simulink model "BaseEngineController_LS"  (Simulink 7.7)
settings: Solver=FixedStepDiscrete  StartTime=0.0  StopTime=10.0  RelTol=1e-3
PreLoadFcn:
  | try, eval([bdroot '_setup']); catch, eval('model_setup', ''); end
InitFcn:
  | try, eval([bdroot '_setup']); catch, eval('model_setup', ''); end
undefined symbols (not defined in the file): ECU555, High, motohawk_build_version, motohawk_trunc_name, motohawk_vardec_config_group, motohawk_vardec_path, True
libraries: MotoHawk_lib x1418, motohawk_control_primitives_lib x183, motohawk_engine_lib x32, simulink x21, motohawk_annotations_lib x9, AutoDoc_lib x8, simulink_extras x4, motohawk_ccp_examples_lib x1, motohawk_control_primitives_motoshare_lib x1
(part 7 of 27)

== system BaseEngineController_LS/Foreground/Control/VirtualSensors/FuelLevel ==
  note: Fuel Level Processed
      | - Detect Refuel Event and immediatly go to new refuled value
      | - If not a refuel event, then filter fuel level at high filter time constant (maybe lower the filter value when vehicle speed is higher), this captures parked on driveway scenario
  Sensors : Inport
  Raw Processed : Inport  Port=2
  Bus Selector : BusSelector  OutputSignals=NonLinearSensors.Fuel_Lvl_Raw
  Bus Selector1 : BusSelector  OutputSignals=TimeSinceKeyOn,VSPD_Final
  First Order Low Pass : motohawk_control_primitives_lib/First Order Low Pass  SystemSampleTime=-1
  FuelLevelWrite : Subsystem  TreatAsAtomicUnit=on
  Logical Operator : Logic  Operator=NOT  AllPortsSameDT=off  OutDataTypeStr=boolean
  Logical Operator1 : Logic  Operator=OR  AllPortsSameDT=off  OutDataTypeStr=boolean
  MinMax : MinMax  Function=max  Inputs=2  SaturateOnIntegerOverflow=on  InputSameDT=on
  Product : Product  Inputs=*/  SaturateOnIntegerOverflow=on  InputSameDT=on  OutDataTypeStr=Inherit: Same as first input
  RefuelEvent : Subsystem
  Switch2 : Switch  Criteria=u2 ~= 0
  Switch3 : Switch  Criteria=u2 ~= 0
  motohawk_calibration2 : MotoHawk_lib/Calibration & Probing Blocks/motohawk_calibration  nam='FuelLevel_FuelEevntAlpha'  val=1  storage=Calibration  show_more=on  name_source=Use Parameter  data_type=Inherit from 'Default Value'  read_level=1  write_level=1  ovr_cals=on  view_as=Number  enum_struct={'Disabled', 'Enabled'}  vector_style=Wide Row  use_help_units=on  help='Fuel event alpha'  units='alpha'  use_header_enum=off  row_header_enum={}  col_header_enum={}  use_min_max=on  min_val=0  max_val=inf  use_precision=off  precision=''  gain=1  offset=0  exp=1  use_mototune_group=off  mototune_group=motohawk_vardec_path(gcb)
  motohawk_data_def : MotoHawk_lib/Data Storage Blocks/motohawk_data_def  nam='FuelLvl_NVM'  container_nam=''  data=0  typ=double  struct_nam='MyStruct'  storage=NonVolatile  outputRef=off  use_vardec=off  window=Calibration  read_level=1  write_level=1  ovr_cals=on  view_as=Number  enum_struct={'Disabled', 'Enabled'}  vector_style=Wide Row  use_help_units=off  help=''  units=''  use_header_enum=off  row_header_enum=''  col_header_enum=''  use_min_max=on  min_val=-inf  max_val=inf  use_precision=off  precision=''  gain=1  offset=0  exp=1  use_mototune_group=off  mototune_group=motohawk_vardec_path(gcb)  eval_name=MyData  data_stores=motohawk_sfun_data_def_data_stores  struct_instances=motohawk_sfun_data_def_struct_instances  vardecs=motohawk_sfun_data_def_vardecs
  motohawk_data_read : MotoHawk_lib/Data Storage Blocks/motohawk_data_read  source=Lookup By Name  structure=Scalar  operation=Read scalar from location by index  sz_vec=4  sz_row=2  sz_col=3  typ=double  nam='FuelLvl_NVM'  checkNull=on  struct_inst_name='MyData'  struct_nam='MyStruct'
  motohawk_delta_time : MotoHawk_lib/Extra Development Blocks/motohawk_delta_time  samp_time=-1  init_val=0  mode=Seconds (double)
  motohawk_probe : MotoHawk_lib/Calibration & Probing Blocks/motohawk_probe  nam='FuelLvl_NVM_Prb'  show_more=off  name_source=Use Parameter  read_level=1  view_as=Number  enum_struct={'Disabled', 'Enabled'}  vector_style=Wide Row  use_help_units=off  help=''  units=''  use_header_enum=off  row_header_enum={}  col_header_enum={}  use_precision=off  precision=''  gain=1  offset=0  exp=1  use_mototune_group=off  mototune_group=motohawk_vardec_path(gcb)
  motohawk_probe1 : MotoHawk_lib/Calibration & Probing Blocks/motohawk_probe  nam='FuelLvl_Fin'  show_more=off  name_source=Use Parameter  read_level=1  view_as=Number  enum_struct={'Disabled', 'Enabled'}  vector_style=Wide Row  use_help_units=off  help=''  units=''  use_header_enum=off  row_header_enum={}  col_header_enum={}  use_precision=off  precision=''  gain=1  offset=0  exp=1  use_mototune_group=off  mototune_group=motohawk_vardec_path(gcb)
  motohawk_table_2d : MotoHawk_lib/Lookup Tables/motohawk_table_2d  SystemSampleTime=-1  nam='FuelLevel_FiltConst'  row_nam=''  col_nam=''  row_breakpoint_data=ones(1,7)  col_breakpoint_data=ones(1,7)  table_data=ones(7)  show_more=on  row_bp_data_type=Inherit from 'Row Breakpoint Data'  col_bp_data_type=Inherit from 'Column Breakpoint Data'  bp_storage=Constant  table_data_type=Inherit from 'Table Data'  storage=NonAdaptive  read_level=1  write_level=1  ovr_cals=on  use_help=on  help='FuelLevel_FiltConst'  row_bp_units='sec'  col_bp_units='mph'  table_units='sec'  use_min_max=on  row_bp_min_val=0  row_bp_max_val=inf  col_bp_min_val=0  col_bp_max_val=inf  min_val=0  max_val=inf  use_precision=off  use_row_breakpoint=off  rb_precision=''  rb_gain=1  rb_offset=0  rb_exp=1  use_col_breakpoint=off  cb_precision=''  cb_gain=1  cb_offset=0  cb_exp=1  use_table=off  t_precision=''  t_gain=1  t_offset=0  t_exp=1  use_links=off  row_input_name=''  col_input_name=''  output_name=''  use_mototune_group=off  mototune_group=motohawk_vardec_path(gcb)
  Fuel Lvl Final : Outport
  wires:
  Sensors/1 -> Bus Selector/1
  Raw Processed/1 -> Bus Selector1/1
  First Order Low Pass/1 -> Fuel Lvl Final/1, motohawk_probe1/1, FuelLevelWrite/1(FuelLevelFilt)
  motohawk_delta_time/1 -> Product/1, MinMax/1
  MinMax/1 -> Product/2
  motohawk_table_2d/1 -> MinMax/2
  Bus Selector1/2 -> motohawk_table_2d/2  "<VSPD_Final>"
  Bus Selector/1 -> RefuelEvent/1(FuelRaw), [FuelLevel]  "<Fuel_Lvl_Raw>"
  Bus Selector1/1 -> RefuelEvent/2(TimeSinceKeyOn), motohawk_table_2d/1  "<TimeSinceKeyOn>"
  RefuelEvent/2(RefuelEventDR) -> Switch2/2, [FuelLevelDR]
  motohawk_data_read/1 -> Switch2/3, motohawk_probe/1
  [FuelLevel] -> Switch2/1
  RefuelEvent/1(RefuelEvent) -> [RefuelEvent]
  [FuelLevelDR] -> Logical Operator/1
  [RefuelEvent] -> Logical Operator1/2
  Logical Operator/1 -> Logical Operator1/1
  Logical Operator1/1 -> Switch3/2
  motohawk_calibration2/1 -> Switch3/1
  Switch2/1 -> First Order Low Pass/1
  Product/1 -> Switch3/3
  Switch3/1 -> First Order Low Pass/2
  [FuelLevelDR] -> FuelLevelWrite/Enable

== system BaseEngineController_LS/Foreground/Control/VirtualSensors/LoadBasedCalcs ==
  RAW : Inport
  Bus Selector : BusSelector  OutputSignals=LinearSensors.MAP_Angular,RPM
  Engine Steady-State Flag : Subsystem  Description=|  AncestorBlock=motohawk_engine_lib/Engine Steady-State Flag  mask(Steady-State Engine Operation){samp_time=-1, group=motohawk_vardec_path(gcb)}
      | /* Name: SSTorqueFilterConst Unit:sec ClassID:VAR StorageID:FLASH Access:RW4+RW3+NA2+NA1 TypeID:UINT2            
      |    Gain:0.001 Min:0.00 Max:65.54 Format:4.2 UpdateID:REMOTE Group:"Engine Control | States" Help:"First-order "  
      |    "filter time constant used to filter torque. This value must be less than SSTorqueTol from unfiltered torque "
      |    "before the steady-state flag can be enabled." VardecSig:6C */                                                
      |                                                                                                                  
      | /* Name: SSRPMFilterConst Unit:sec ClassID:VAR StorageID:FLASH Access:RW4+RW3+NA2+NA1 TypeID:UINT2               
      |    Gain:0.001 Min:0.00 Max:65.54 Format:4.2 UpdateID:REMOTE Group:"Engine Control | States" Help:"First-order "  
      |    "filter time constant used to filter torque. This value must be less than SSRPMTol from unfiltered torque "   
      |    "before the steady-state flag can be enabled." VardecSig:6C */                                                
      |                                                                                                                  
      | /* Name: SSTorqueTol Unit:N.m ClassID:VAR StorageID:FLASH Access:RW4+RW3+NA2+NA1 TypeID:UINT2 Gain:0.001         
      |    Min:0.00 Max:65.54 Format:4.2 UpdateID:REMOTE Group:"Engine Control | States" Help:"Tolerance within which "  
      |    "the difference between filtered and unfiltered torque must lie before the steady-state flag can be "         
      |    "enabled." VardecSig:6C */                                                                                    
      |                                                                                                                  
      | /* Name: SSRPMTol Unit:RPM ClassID:VAR StorageID:FLASH Access:RW4+RW3+NA2+NA1 TypeID:UINT2 Gain:0.01             
      |    Min:0.00 Max:655.35 Format:4.2 UpdateID:REMOTE Group:"Engine Control | States" Help:"Tolerance within which " 
      |    "the difference between filtered and unfiltered RPM must lie before the steady-state flag can be enabled."    
      |    VardecSig:6C */
      mask prompts: samp_time "Sample Time [s]:"; group "MotoTune Group String"
      mask help:
      | This block determines whether or not the engine has achieved steady-state operation. It accomplishes this by applying a first-order low-pass filter to the indicated torque and RPM inputs. The filetrcoeficeints are individually calibratable for each. Once both the filtered torque and RPM values are within the calibratable toleraance of the input values, engine operation is assumed to be steady-state.
      |
      | If 'Sample Time' is -1, then extra code and RAM will be generated to dynamically calculate dt.
      mask Display:
      | patch([0 0 1 1], [0 0.075 0.075 0], [230/255 0/255 0/255])
      | patch([0 0 1 1], [0.025 0.05 0.05 0.025], [150/255 0/255 0/255])
      | patch([0 0 1 1], [0 0.025 0.025 0], [0/255 0/255 0/255])
      | 
      | disp('ENGINE\nSTEADY-STATE\nDETERMINATION')
  motohawk_probe : MotoHawk_lib/Calibration & Probing Blocks/motohawk_probe  nam='SSEng'  show_more=off  name_source=Use Parameter  read_level=1  view_as=Number  enum_struct={'Disabled', 'Enabled'}  vector_style=Wide Row  use_help_units=off  help=''  units=''  use_header_enum=off  row_header_enum={}  col_header_enum={}  use_precision=off  precision=''  gain=1  offset=0  exp=1  use_mototune_group=off  mototune_group=motohawk_vardec_path(gcb)
  SSEng : Outport
  wires:
  Engine Steady-State Flag/1(SSEngOpr [bool]) -> SSEng/1, motohawk_probe/1  "SSEng"
  RAW/1 -> Bus Selector/1
  Bus Selector/1 -> Engine Steady-State Flag/1(Load)  "<MAP_Angular>"
  Bus Selector/2 -> Engine Steady-State Flag/2(RPM)  "<RPM>"

== system BaseEngineController_LS/Foreground/Control/VirtualSensors/Raw Indexes ==
  Raw : Inport
  RawProcessed : Inport  Port=2
  ACPres Index : Subsystem
  Bus Creator1 : BusCreator  Inputs=21
  Bus Selector : BusSelector  OutputSignals=TPS
  Bus Selector1 : BusSelector  OutputSignals=LinearSensors.ACPres
  Bus Selector2 : BusSelector  OutputSignals=LinearSensors.SysVolt
  Bus Selector3 : BusSelector  OutputSignals=LinearSensors.MAP_Angular
  Bus Selector4 : BusSelector  OutputSignals=VSPD_Final
  Bus Selector5 : BusSelector  OutputSignals=NonLinearSensors.CAT
  Bus Selector6 : BusSelector  OutputSignals=RPM
  Bus Selector7 : BusSelector  OutputSignals=NonLinearSensors.IAT
  Bus Selector8 : BusSelector  OutputSignals=NonLinearSensors.ECT
  Bus Selector9 : BusSelector  OutputSignals=LinearSensors.FuelSense
  CAT Index : Subsystem
  ECT Index : Subsystem
  IAT Indexes : Subsystem
  MAP Indexes : Subsystem
  OXY Index : Subsystem
  RPM Indexes : Subsystem
  SysVolt Index : Subsystem
  TPS Indexes : Subsystem
  VSPD Index : Subsystem
  RawIndexes : Outport
  wires:
  RPM Indexes/1(RPM05Idx) -> Bus Creator1/1  "RPM05Idx"
  RPM Indexes/2(RPM09Idx) -> Bus Creator1/2  "RPM09Idx"
  TPS Indexes/1(TPS09Idx) -> Bus Creator1/4  "TPS09Idx"
  Bus Selector7/1 -> IAT Indexes/1(IAT)  "<IAT>"
  ECT Index/1(ECT05Idx) -> Bus Creator1/5  "ECT05Idx"
  Bus Selector8/1 -> ECT Index/1(ECT)  "<ECT>"
  Bus Creator1/1 -> RawIndexes/1  "RawIndexes"
  Bus Selector6/1 -> RPM Indexes/1(RPM)  "<RPM>"
  Raw/1 -> Bus Selector6/1, Bus Selector8/1, Bus Selector7/1, Bus Selector2/1, Bus Selector1/1, Bus Selector3/1, Bus Selector5/1, Bus Selector9/1
  Bus Selector2/1 -> SysVolt Index/1(SysVolt)  "<SysVolt>"
  RPM Indexes/3(RPM17Idx) -> Bus Creator1/3  "RPM17Idx"
  Bus Selector1/1 -> ACPres Index/1(ACPres)  "<ACPres>"
  Bus Selector3/1 -> MAP Indexes/1(MAP)  "<MAP_Angular>"
  Bus Selector4/1 -> VSPD Index/1(VSPD)  "<VSPD_Final>"
  Bus Selector5/1 -> CAT Index/1(CAT)  "<CAT>"
  Bus Selector9/1 -> OXY Index/1(CAT)  "<FuelSense>"
  RawProcessed/1 -> Bus Selector/1, Bus Selector4/1
  Bus Selector/1 -> TPS Indexes/1(TPSPcnt)  "<TPS>"
  ECT Index/3(ECT09Idx) -> Bus Creator1/7  "ECT09Idx"
  ECT Index/2(ECT07Idx) -> Bus Creator1/6  "ECT07Idx"
  IAT Indexes/1(IAT05Idx) -> Bus Creator1/8  "IAT05Idx"
  IAT Indexes/2(IAT07Idx) -> Bus Creator1/9  "IAT07Idx"
  IAT Indexes/3(IAT17Idx) -> Bus Creator1/10  "IAT17Idx"
  SysVolt Index/1(SysVolt09Idx) -> Bus Creator1/11  "SysVolt09Idx"
  ACPres Index/1(ACPres05Idx) -> Bus Creator1/12  "ACPres05Idx"
  ACPres Index/2(ACPres07Idx) -> Bus Creator1/13  "ACPres07Idx"
  OXY Index/1(OXY05Idx) -> Bus Creator1/21  "OXY05Idx"
  CAT Index/1(CAT05Idx) -> Bus Creator1/20  "CAT05Idx"
  VSPD Index/3(VSPD17Idx) -> Bus Creator1/19  "VSPD17Idx"
  VSPD Index/2(VSPD07Idx) -> Bus Creator1/18  "VSPD07Idx"
  VSPD Index/1(VSPD09Idx) -> Bus Creator1/17  "VSPD09Idx"
  MAP Indexes/1(MAP05Idx) -> Bus Creator1/14  "MAP05Idx"
  MAP Indexes/2(MAP09Idx) -> Bus Creator1/15  "MAP09Idx"
  MAP Indexes/3(MAP17Idx) -> Bus Creator1/16  "MAP17Idx"

== system BaseEngineController_LS/Foreground/Control/VirtualSensors/RawProcessed ==
  Raw : Inport
  Indexes : Inport  Port=2
  APP  Sensor Arbitration1 : Subsystem
      mask Display:
      | patch([0 0 1 1], [0 0.075 0.075 0], [230/255 0/255 0/255])
      | patch([0 0 1 1], [0.025 0.05 0.05 0.025], [150/255 0/255 0/255])
      | patch([0 0 1 1], [0 0.025 0.025 0], [0/255 0/255 0/255])
      | 
      | disp('APPSensor\nArbitration');
  Base TPS Request : Subsystem  TreatAsAtomicUnit=on
  Bus Creator : BusCreator  Inputs=2
  Bus Creator2 : BusCreator  Inputs=17
  Bus Selector1 : BusSelector  OutputSignals=PotSensors.TPS2
  Bus Selector10 : BusSelector  OutputSignals=PotSensors.TPS1
  Bus Selector11 : BusSelector  OutputSignals=CAN.O2_BankA,CAN.O2_BankB
  Bus Selector12 : BusSelector  OutputSignals=RPM
  Bus Selector13 : BusSelector  OutputSignals=Digital.VSPD,CAN.GPS_BUS.GPS_Speed_Dir.GPS_Speed,CAN.GPS_BUS.GPS_Date_Time.GPS_Valid
  Bus Selector2 : BusSelector  OutputSignals=RPMInst
  Bus Selector3 : BusSelector  OutputSignals=LinearSensors.FuelPres,LinearSensors.Map_Time
  Bus Selector4 : BusSelector  OutputSignals=PotSensors.APP1,PotSensors.APP2
  Bus Selector5 : BusSelector  OutputSignals=NonLinearSensors.ECT_Raw
  Bus Selector6 : BusSelector  OutputSignals=TPS09Idx
  Bus Selector7 : BusSelector  OutputSignals=NonLinearSensors.IAT_Raw
  Bus Selector8 : BusSelector  OutputSignals=RPM,Digital.ClutchSw
  Bus Selector9 : BusSelector  OutputSignals=VSPD17Idx
  Capture ECT At Startup : Subsystem  TreatAsAtomicUnit=on  mask(Capture Signal At Startup){nam='ECT_KeyUp', count=5, units='C', grp=motohawk_vardec_path(gcb)}
      mask prompts: nam "Signal Name"; count "Number Of Samples To Average"; grp "MotoTune GroupString Name"
      mask init:
      | lbl = sprintf('CAPTURE IN STALL\nAverage of\nfirst %d samples', count);
      mask Display:
      | patch([0 0 1 1], [0 0.075 0.075 0], [230/255 0/255 0/255])
      | patch([0 0 1 1], [0.025 0.05 0.05 0.025], [150/255 0/255 0/255])
      | patch([0 0 1 1], [0 0.025 0.025 0], [0/255 0/255 0/255])
      | 
      | disp(lbl);
  Capture IAT At Startup : Subsystem  TreatAsAtomicUnit=on  mask(Capture Signal At Startup){nam='IAT_KeyUp', count=5, units='C', grp='Sensors | IAT'}
      mask prompts: nam "Signal Name"; count "Number Of Samples To Average"; grp "MotoTune GroupString Name"
      mask init:
      | lbl = sprintf('CAPTURE IN STALL\nAverage of\nfirst %d samples', count);
      mask Display:
      | patch([0 0 1 1], [0 0.075 0.075 0], [230/255 0/255 0/255])
      | patch([0 0 1 1], [0.025 0.05 0.05 0.025], [150/255 0/255 0/255])
      | patch([0 0 1 1], [0 0.025 0.025 0], [0/255 0/255 0/255])
      | 
      | disp(lbl);
  CutThrottle APP Limiting : Subsystem
      mask Display:
      | patch([0 0 1 1], [0 0.075 0.075 0], [230/255 0/255 0/255])
      | patch([0 0 1 1], [0.025 0.05 0.05 0.025], [150/255 0/255 0/255])
      | patch([0 0 1 1], [0 0.025 0.025 0], [0/255 0/255 0/255])
      | 
      | disp('');
  Data Type Conversion : DataTypeConversion  OutDataTypeStr=double
  Engine Accel : Subsystem
  EngineState : Subsystem
      mask Display: disp('ENGINE STATE\nDETERMINATION\n\n1 - Stall\n2 - Crank\n3 - Run');
  Fuel Delta Pressure Calculation : Subsystem
      mask Display:
      | patch([0 0 1 1], [0 0.075 0.075 0], [230/255 0/255 0/255])
      | patch([0 0 1 1], [0.025 0.05 0.05 0.025], [150/255 0/255 0/255])
      | patch([0 0 1 1], [0 0.025 0.025 0], [0/255 0/255 0/255])
      | 
      | disp('Fuel Pressure \n Across Injectors');
  Gear Estimator : Subsystem
  O2 De-lag : Subsystem
  Stall : motohawk_control_primitives_lib/CompareTo  SystemSampleTime=-1  op===  val=1
  TPS  Sensor Arbitration : Subsystem
      mask Display:
      | patch([0 0 1 1], [0 0.075 0.075 0], [230/255 0/255 0/255])
      | patch([0 0 1 1], [0.025 0.05 0.05 0.025], [150/255 0/255 0/255])
      | patch([0 0 1 1], [0 0.025 0.025 0], [0/255 0/255 0/255])
      | 
      | disp('TPS Sensor\nArbitration');
  Time Since Key On : Subsystem
  Time Since Run : Subsystem
  Time Since Stall : Subsystem
  VSPD_Selector : Subsystem
  motohawk_data_read : MotoHawk_lib/Data Storage Blocks/motohawk_data_read  source=Lookup By Name  structure=Scalar  operation=Read entire data structure at once  sz_vec=4  sz_row=2  sz_col=3  typ=uint8  nam='EngineState'  checkNull=on  struct_inst_name='Struct1'  struct_nam='MyStruct'
  motohawk_probe : MotoHawk_lib/Calibration & Probing Blocks/motohawk_probe  nam='APPPcnt'  show_more=on  name_source=Use Parameter  read_level=1  view_as=Number  enum_struct={'Disabled', 'Enabled'}  vector_style=Wide Row  use_help_units=on  help='APP used in controller (after power curve and CutThrottle limiting'  units='%'  use_header_enum=off  row_header_enum={}  col_header_enum={}  use_precision=on  precision=''  gain=1  offset=0  exp=1  use_mototune_group=on  mototune_group=motohawk_vardec_path(gcb)
  RawProcessed : Outport
  wires:
  Base TPS Request/3(APP Idx) -> Bus Creator2/6  "APPIdx"
  Bus Selector7/1 -> Capture IAT At Startup/1(Signal_In)  "<IAT_Raw>"
  Capture IAT At Startup/1(Signal_KeyUp) -> Bus Creator2/15  "IAT_KeyUp"
  Bus Selector2/1 -> EngineState/1(RPM)  "<RPMInst>"
  Bus Selector12/1 -> Engine Accel/1(RPM)  "<RPM>"
  EngineState/1(State) -> Bus Creator2/1  "EngineState"
  Base TPS Request/1(ETCReqFilt) -> Bus Creator2/4  "ETCRequest"
  Engine Accel/1(RPM Accel) -> Bus Creator2/9  "RPM_Accel"
  Bus Creator2/1 -> RawProcessed/1  "RawProcessed"
  Raw/1 -> Bus Selector11/1, Bus Selector12/1, Bus Selector10/1, Bus Selector5/1, Bus Selector7/1, Bus Selector8/1, Bus Selector13/1, Bus Selector1/1, Bus Selector3/1, Bus Selector4/1, Bus Selector2/1
  Bus Selector10/1 -> TPS  Sensor Arbitration/1(TPS1)  "<TPS1>"
  Bus Selector1/1 -> TPS  Sensor Arbitration/2(TPS2)  "<TPS2>"
  TPS  Sensor Arbitration/1(TPS) -> Data Type Conversion/1  "TPS"
  Bus Selector5/1 -> Capture ECT At Startup/1(Signal_In)  "<ECT_Raw>"
  motohawk_data_read/1 -> Stall/1
  Stall/1 -> Capture IAT At Startup/Enable, Capture ECT At Startup/Enable
  Capture ECT At Startup/1(Signal_KeyUp) -> Bus Creator2/11  "ECT_KeyUp"
  Base TPS Request/2(ETCReqRaw) -> Bus Creator2/5  "ETCReqRaw"
  Time Since Stall/1(Time) -> Bus Creator2/12  "TimeSinceStall"
  Time Since Run/1(Time) -> Bus Creator2/13  "TimeSinceRun"
  Bus Selector6/1 -> Base TPS Request/2(TPS_Idx)  "<TPS09Idx>"
  Time Since Key On/1(Time) -> Bus Creator2/14  "TimeSinceKeyOn"
  Bus Creator/1 -> Bus Creator2/8  "O2Delagged"
  O2 De-lag/1(O2BankADelagged) -> Bus Creator/1  "O2BankADelagged"
  O2 De-lag/2(O2BankBDelagged) -> Bus Creator/2  "O2BankBDelagged"
  Bus Selector3/1 -> Fuel Delta Pressure Calculation/1(FuelPressure)  "<FuelPres>"
  Bus Selector3/2 -> Fuel Delta Pressure Calculation/2("MAP ")  "<Map_Time>"
  Fuel Delta Pressure Calculation/1("FuelDeltaPressure ") -> Bus Creator2/7  "FuelDeltaPressure"
  CutThrottle APP Limiting/1(APP_out [%]) -> Bus Creator2/2, motohawk_probe/1, Base TPS Request/1(APP Pcnt)  "APPPcnt"
  Bus Selector4/1 -> APP  Sensor Arbitration1/1(APP1), Bus Creator2/3  "<APP1>"
  Bus Selector4/2 -> APP  Sensor Arbitration1/2(APP2)  "<APP2>"
  APP  Sensor Arbitration1/1(APP) -> CutThrottle APP Limiting/1(APP_in [%])  "APP1"
  Indexes/1 -> Bus Selector6/1, Bus Selector9/1
  Gear Estimator/1(Gear) -> Bus Creator2/16  "GearEst"
  Bus Selector8/1 -> Gear Estimator/1(RPM)  "<RPM>"
  Bus Selector8/2 -> Gear Estimator/3(ClutchSW)  "<ClutchSw>"
  Bus Selector9/1 -> Base TPS Request/3(VSPD17Idx)  "<VSPD17Idx>"
  VSPD_Selector/1(VSPD_Final) -> Bus Creator2/17, Gear Estimator/2(VSPD)  "VSPD_Final"
  Bus Selector13/2 -> VSPD_Selector/2(VSPD_GPS)  "<GPS_Speed>"
  Bus Selector13/3 -> VSPD_Selector/3(VSPD_GPSValid)  "<GPS_Valid>"
  Bus Selector13/1 -> VSPD_Selector/1(VSPD_Dig)  "<VSPD>"
  Data Type Conversion/1 -> Bus Creator2/10  "TPS"
  Bus Selector11/1 -> O2 De-lag/1(O2_BankA)  "<O2_BankA>"
  Bus Selector11/2 -> O2 De-lag/2(O2_BankB)  "<O2_BankB>"

== system BaseEngineController_LS/Foreground/Control/VirtualSensors/Virtual Indexes ==
  AirCalcs : Inport
  RawProcessed : Inport  Port=2
  Bus Creator2 : BusCreator  Inputs=6
  Bus Selector3 : BusSelector  OutputSignals=MAFPort
  Bus Selector4 : BusSelector  OutputSignals=ECT_KeyUp
  Bus Selector5 : BusSelector  OutputSignals=RPM_Accel
  Bus Selector6 : BusSelector  OutputSignals=APP1
  Bus Selector7 : BusSelector  OutputSignals=TimeSinceRun
  Bus Selector8 : BusSelector  OutputSignals=IAT_KeyUp
  ECT_KeyUp : Subsystem
  IAT_KeyUp : Subsystem
  MAFPortIndex : Subsystem
  motohawk_prelookup : MotoHawk_lib/Lookup Tables/motohawk_prelookup  nam='RPMAccel17'  breakpoint_data=ones(1,17)  show_more=on  data_type=Inherit from 'Table Data'  storage=Constant  read_level=1  write_level=1  ovr_cals=on  use_help=on  help=''  units=''  use_min_max=off  min_val=-inf  max_val=inf  use_precision=on  precision=''  gain=1  offset=0  exp=1  use_links=off  input_name=''  use_mototune_group=on  mototune_group=motohawk_vardec_path(gcb)
  motohawk_prelookup1 : MotoHawk_lib/Lookup Tables/motohawk_prelookup  nam='App05'  breakpoint_data=[0 50 70 90 100]  show_more=on  data_type=Inherit from 'Table Data'  storage=Constant  read_level=1  write_level=1  ovr_cals=on  use_help=on  help=''  units=''  use_min_max=off  min_val=-inf  max_val=inf  use_precision=on  precision=''  gain=1  offset=0  exp=1  use_links=off  input_name=''  use_mototune_group=on  mototune_group=motohawk_vardec_path(gcb)
  motohawk_prelookup2 : MotoHawk_lib/Lookup Tables/motohawk_prelookup  nam='TimeSinceRun09'  breakpoint_data=[0 2 4 6 10 15 20 30 45]  show_more=on  data_type=Inherit from 'Table Data'  storage=Constant  read_level=1  write_level=1  ovr_cals=on  use_help=on  help=''  units=''  use_min_max=off  min_val=-inf  max_val=inf  use_precision=on  precision=''  gain=1  offset=0  exp=1  use_links=off  input_name=''  use_mototune_group=on  mototune_group=motohawk_vardec_path(gcb)
  VirtualIndexes : Outport
  wires:
  Bus Creator2/1 -> VirtualIndexes/1  "Virtual Indexes"
  AirCalcs/1 -> Bus Selector3/1
  Bus Selector3/1 -> MAFPortIndex/1(MAFPort)  "<MAFPort>"
  Bus Selector4/1 -> ECT_KeyUp/1(ECT_KeyUp)  "<ECT_KeyUp>"
  RawProcessed/1 -> Bus Selector4/1, Bus Selector5/1, Bus Selector6/1, Bus Selector7/1, Bus Selector8/1
  Bus Selector5/1 -> motohawk_prelookup/1  "<RPM_Accel>"
  Bus Selector6/1 -> motohawk_prelookup1/1  "<APP1>"
  Bus Selector7/1 -> motohawk_prelookup2/1  "<TimeSinceRun>"
  Bus Selector8/1 -> IAT_KeyUp/1(IAT_KeyUp)  "<IAT_KeyUp>"
  MAFPortIndex/1(MAFPort05Idx) -> Bus Creator2/1  "MAFPort05Idx"
  ECT_KeyUp/1(ECT_KeyUp09Idx) -> Bus Creator2/2  "ECTKeyUp09Idx"
  motohawk_prelookup/1 -> Bus Creator2/3  "RPMAccel17Idx"
  motohawk_prelookup1/1 -> Bus Creator2/4  "App05Idx"
  motohawk_prelookup2/1 -> Bus Creator2/5  "TimeSinceRun09"
  IAT_KeyUp/1(IAT_KeyUp09Idx) -> Bus Creator2/6  "IATKeyUp09Idx"

== system BaseEngineController_LS/Foreground/Inputs/CAN/AEM GPS ==
  Bus Creator : BusCreator  Inputs=7
  Bus Creator1 : BusCreator  Inputs=2
  Bus Creator2 : BusCreator
  Bus Creator3 : BusCreator  Inputs=3
  Data Type Conversion{,1..5,8} (7 alike) : DataTypeConversion  OutDataTypeStr=uint8
  Read CAN Message : MotoHawk_lib/CAN Blocks/Read CAN Message  nam='CAN_1'  bus=-2  msg=CANRx_AEM_GPS_DATE_TIME  queue=1  slot=''  valid=off  stale=on  labelwires=off
  Read CAN Message1 : MotoHawk_lib/CAN Blocks/Read CAN Message  nam='CAN_1'  bus=-2  msg=CANRx_AEM_GPS_LAT_LONG  queue=1  slot=''  valid=off  stale=on  labelwires=off
  Read CAN Message2 : MotoHawk_lib/CAN Blocks/Read CAN Message  nam='CAN_1'  bus=-2  msg=CANRx_AEM_GPS_SPEED_DIRECTION  queue=1  slot=''  valid=off  stale=on  labelwires=off
  Relational Operator : RelationalOperator  OutDataTypeStr=boolean
  Relational Operator1 : RelationalOperator  OutDataTypeStr=boolean
  Relational Operator2 : RelationalOperator  OutDataTypeStr=boolean
  motohawk_calibration : MotoHawk_lib/Calibration & Probing Blocks/motohawk_calibration  nam='GPS_DateTime_Timeout'  val=100  storage=Calibration  show_more=on  name_source=Use Parameter  data_type=uint16  read_level=1  write_level=1  ovr_cals=on  view_as=Number  enum_struct={'Disabled', 'Enabled'}  vector_style=Wide Row  use_help_units=on  help=''  units='ms'  use_header_enum=off  row_header_enum={}  col_header_enum={}  use_min_max=off  min_val=-inf  max_val=inf  use_precision=off  precision=''  gain=1  offset=0  exp=1  use_mototune_group=off  mototune_group=motohawk_vardec_path(gcb)
  motohawk_calibration1 : MotoHawk_lib/Calibration & Probing Blocks/motohawk_calibration  nam='GPS_LatLong_Timeout'  val=100  storage=Calibration  show_more=on  name_source=Use Parameter  data_type=uint16  read_level=1  write_level=1  ovr_cals=on  view_as=Number  enum_struct={'Disabled', 'Enabled'}  vector_style=Wide Row  use_help_units=on  help=''  units='ms'  use_header_enum=off  row_header_enum={}  col_header_enum={}  use_min_max=off  min_val=-inf  max_val=inf  use_precision=off  precision=''  gain=1  offset=0  exp=1  use_mototune_group=off  mototune_group=motohawk_vardec_path(gcb)
  motohawk_calibration2 : MotoHawk_lib/Calibration & Probing Blocks/motohawk_calibration  nam='GPS_SpeedDir_Timeout'  val=100  storage=Calibration  show_more=on  name_source=Use Parameter  data_type=uint16  read_level=1  write_level=1  ovr_cals=on  view_as=Number  enum_struct={'Disabled', 'Enabled'}  vector_style=Wide Row  use_help_units=on  help=''  units='ms'  use_header_enum=off  row_header_enum={}  col_header_enum={}  use_min_max=off  min_val=-inf  max_val=inf  use_precision=off  precision=''  gain=1  offset=0  exp=1  use_mototune_group=off  mototune_group=motohawk_vardec_path(gcb)
  motohawk_fault_def1 : MotoHawk_lib/Fault Management Blocks/motohawk_fault_def  nam='GPS_LatLong_Timeout'  mode=Enabled  id=[]  x=1  y=2  input_suspected=on  indeterminate=off  increment_xy=on  downsample_count=1  ovr_cals=on  ovr_actions=on  show_actions=on  action1_name=''  action1_cond=(None)  action2_name=''  action2_cond=(None)  action3_name=''  action3_cond=(None)  action4_name=''  action4_cond=(None)
  motohawk_fault_def2 : MotoHawk_lib/Fault Management Blocks/motohawk_fault_def  nam='GPS_DateTime_Timeout'  mode=Enabled  id=[]  x=1  y=2  input_suspected=on  indeterminate=off  increment_xy=on  downsample_count=1  ovr_cals=on  ovr_actions=on  show_actions=on  action1_name=''  action1_cond=(None)  action2_name=''  action2_cond=(None)  action3_name=''  action3_cond=(None)  action4_name=''  action4_cond=(None)
  motohawk_fault_def4 : MotoHawk_lib/Fault Management Blocks/motohawk_fault_def  nam='GPS_SpeedDir_Timeout'  mode=Enabled  id=[]  x=1  y=2  input_suspected=on  indeterminate=off  increment_xy=on  downsample_count=1  ovr_cals=on  ovr_actions=on  show_actions=on  action1_name=''  action1_cond=(None)  action2_name=''  action2_cond=(None)  action3_name=''  action3_cond=(None)  action4_name=''  action4_cond=(None)
  motohawk_probe : MotoHawk_lib/Calibration & Probing Blocks/motohawk_probe  nam='GPS_Valid_Prb'  show_more=off  name_source=Use Parameter  read_level=1  view_as=Number  enum_struct={'Disabled', 'Enabled'}  vector_style=Wide Row  use_help_units=off  help=''  units=''  use_header_enum=off  row_header_enum={}  col_header_enum={}  use_precision=off  precision=''  gain=1  offset=0  exp=1  use_mototune_group=off  mototune_group=motohawk_vardec_path(gcb)
  motohawk_probe1 : MotoHawk_lib/Calibration & Probing Blocks/motohawk_probe  nam='GPS_YearUTC_Prb'  show_more=off  name_source=Use Parameter  read_level=1  view_as=Number  enum_struct={'Disabled', 'Enabled'}  vector_style=Wide Row  use_help_units=off  help=''  units=''  use_header_enum=off  row_header_enum={}  col_header_enum={}  use_precision=off  precision=''  gain=1  offset=0  exp=1  use_mototune_group=off  mototune_group=motohawk_vardec_path(gcb)
  motohawk_probe10 : MotoHawk_lib/Calibration & Probing Blocks/motohawk_probe  nam='GPS_Altitude_Prb'  show_more=off  name_source=Use Parameter  read_level=1  view_as=Number  enum_struct={'Disabled', 'Enabled'}  vector_style=Wide Row  use_help_units=off  help=''  units=''  use_header_enum=off  row_header_enum={}  col_header_enum={}  use_precision=off  precision=''  gain=1  offset=0  exp=1  use_mototune_group=off  mototune_group=motohawk_vardec_path(gcb)
  motohawk_probe11 : MotoHawk_lib/Calibration & Probing Blocks/motohawk_probe  nam='GPS_Course_Prb'  show_more=off  name_source=Use Parameter  read_level=1  view_as=Number  enum_struct={'Disabled', 'Enabled'}  vector_style=Wide Row  use_help_units=off  help=''  units=''  use_header_enum=off  row_header_enum={}  col_header_enum={}  use_precision=off  precision=''  gain=1  offset=0  exp=1  use_mototune_group=off  mototune_group=motohawk_vardec_path(gcb)
  motohawk_probe12 : MotoHawk_lib/Calibration & Probing Blocks/motohawk_probe  nam='GPS_SatelliteCount_Prb'  show_more=off  name_source=Use Parameter  read_level=1  view_as=Number  enum_struct={'Disabled', 'Enabled'}  vector_style=Wide Row  use_help_units=off  help=''  units=''  use_header_enum=off  row_header_enum={}  col_header_enum={}  use_precision=off  precision=''  gain=1  offset=0  exp=1  use_mototune_group=off  mototune_group=motohawk_vardec_path(gcb)
  motohawk_probe2 : MotoHawk_lib/Calibration & Probing Blocks/motohawk_probe  nam='GPS_MonthUTC_Prb'  show_more=off  name_source=Use Parameter  read_level=1  view_as=Number  enum_struct={'Disabled', 'Enabled'}  vector_style=Wide Row  use_help_units=off  help=''  units=''  use_header_enum=off  row_header_enum={}  col_header_enum={}  use_precision=off  precision=''  gain=1  offset=0  exp=1  use_mototune_group=off  mototune_group=motohawk_vardec_path(gcb)
  motohawk_probe3 : MotoHawk_lib/Calibration & Probing Blocks/motohawk_probe  nam='GPS_DayUTC_Prb'  show_more=off  name_source=Use Parameter  read_level=1  view_as=Number  enum_struct={'Disabled', 'Enabled'}  vector_style=Wide Row  use_help_units=off  help=''  units=''  use_header_enum=off  row_header_enum={}  col_header_enum={}  use_precision=off  precision=''  gain=1  offset=0  exp=1  use_mototune_group=off  mototune_group=motohawk_vardec_path(gcb)
  motohawk_probe4 : MotoHawk_lib/Calibration & Probing Blocks/motohawk_probe  nam='GPS_HoursUTC_Prb'  show_more=off  name_source=Use Parameter  read_level=1  view_as=Number  enum_struct={'Disabled', 'Enabled'}  vector_style=Wide Row  use_help_units=off  help=''  units=''  use_header_enum=off  row_header_enum={}  col_header_enum={}  use_precision=off  precision=''  gain=1  offset=0  exp=1  use_mototune_group=off  mototune_group=motohawk_vardec_path(gcb)
  motohawk_probe5 : MotoHawk_lib/Calibration & Probing Blocks/motohawk_probe  nam='GPS_MinutesUTC_Prb'  show_more=off  name_source=Use Parameter  read_level=1  view_as=Number  enum_struct={'Disabled', 'Enabled'}  vector_style=Wide Row  use_help_units=off  help=''  units=''  use_header_enum=off  row_header_enum={}  col_header_enum={}  use_precision=off  precision=''  gain=1  offset=0  exp=1  use_mototune_group=off  mototune_group=motohawk_vardec_path(gcb)
  motohawk_probe6 : MotoHawk_lib/Calibration & Probing Blocks/motohawk_probe  nam='GPS_SecondsUTC_Prb'  show_more=off  name_source=Use Parameter  read_level=1  view_as=Number  enum_struct={'Disabled', 'Enabled'}  vector_style=Wide Row  use_help_units=off  help=''  units=''  use_header_enum=off  row_header_enum={}  col_header_enum={}  use_precision=off  precision=''  gain=1  offset=0  exp=1  use_mototune_group=off  mototune_group=motohawk_vardec_path(gcb)
  motohawk_probe7 : MotoHawk_lib/Calibration & Probing Blocks/motohawk_probe  nam='GPS_Latitude_Prb'  show_more=off  name_source=Use Parameter  read_level=1  view_as=Number  enum_struct={'Disabled', 'Enabled'}  vector_style=Wide Row  use_help_units=off  help=''  units=''  use_header_enum=off  row_header_enum={}  col_header_enum={}  use_precision=off  precision=''  gain=1  offset=0  exp=1  use_mototune_group=off  mototune_group=motohawk_vardec_path(gcb)
  motohawk_probe8 : MotoHawk_lib/Calibration & Probing Blocks/motohawk_probe  nam='GPS_Longitude_Prb'  show_more=off  name_source=Use Parameter  read_level=1  view_as=Number  enum_struct={'Disabled', 'Enabled'}  vector_style=Wide Row  use_help_units=off  help=''  units=''  use_header_enum=off  row_header_enum={}  col_header_enum={}  use_precision=off  precision=''  gain=1  offset=0  exp=1  use_mototune_group=off  mototune_group=motohawk_vardec_path(gcb)
  motohawk_probe9 : MotoHawk_lib/Calibration & Probing Blocks/motohawk_probe  nam='GPS_Speed_Prb'  show_more=off  name_source=Use Parameter  read_level=1  view_as=Number  enum_struct={'Disabled', 'Enabled'}  vector_style=Wide Row  use_help_units=off  help=''  units=''  use_header_enum=off  row_header_enum={}  col_header_enum={}  use_precision=off  precision=''  gain=1  offset=0  exp=1  use_mototune_group=off  mototune_group=motohawk_vardec_path(gcb)
  GPS_BUS : Outport
  wires:
  Read CAN Message/1 -> Relational Operator/1
  motohawk_calibration/1 -> Relational Operator/2
  Relational Operator/1 -> motohawk_fault_def2/1
  Read CAN Message/2 -> motohawk_probe/1, Bus Creator/1  "GPS_Valid"
  Read CAN Message/3 -> Data Type Conversion/1
  Read CAN Message/4 -> Data Type Conversion1/1
  Read CAN Message/5 -> Data Type Conversion2/1
  Read CAN Message/6 -> Data Type Conversion3/1
  Read CAN Message/7 -> Data Type Conversion4/1
  Read CAN Message/8 -> Data Type Conversion5/1
  Read CAN Message1/1 -> Relational Operator1/1
  motohawk_calibration1/1 -> Relational Operator1/2
  Relational Operator1/1 -> motohawk_fault_def1/1
  Read CAN Message1/2 -> motohawk_probe7/1, Bus Creator1/1  "GPS_Latitude"
  Read CAN Message1/3 -> motohawk_probe8/1, Bus Creator1/2  "GPS_Longitude"
  Read CAN Message2/1 -> Relational Operator2/1
  motohawk_calibration2/1 -> Relational Operator2/2
  Relational Operator2/1 -> motohawk_fault_def4/1
  Read CAN Message2/2 -> motohawk_probe9/1, Bus Creator2/1  "GPS_Speed"
  Read CAN Message2/3 -> motohawk_probe10/1, Bus Creator2/2  "GPS_Altitude"
  Read CAN Message2/4 -> motohawk_probe11/1, Bus Creator2/3  "GPS_Course"
  Read CAN Message2/5 -> Data Type Conversion8/1
  Bus Creator/1 -> Bus Creator3/1  "GPS_Date_Time"
  Bus Creator1/1 -> Bus Creator3/2  "GPS_Lat_Long"
  Bus Creator2/1 -> Bus Creator3/3  "GPS_Speed_Dir"
  Bus Creator3/1 -> GPS_BUS/1
  Data Type Conversion/1 -> motohawk_probe1/1, Bus Creator/2  "GPS_YearUTC"
  Data Type Conversion1/1 -> motohawk_probe2/1, Bus Creator/3  "GPS_MonthUTC"
  Data Type Conversion2/1 -> motohawk_probe3/1, Bus Creator/4  "GPS_DayUTC"
  Data Type Conversion3/1 -> motohawk_probe4/1, Bus Creator/5  "GPS_HoursUTC"
  Data Type Conversion4/1 -> motohawk_probe5/1, Bus Creator/6  "GPS_MinutesUTC"
  Data Type Conversion5/1 -> motohawk_probe6/1, Bus Creator/7  "GPS_SecondsUTC"
  Data Type Conversion8/1 -> motohawk_probe12/1, Bus Creator2/4  "GPS_SatelliteCount"
